simulink model "IRControlledSlidingDoor_Test"  (R2016a)
settings: Solver=ode3  SolverMode=SingleTasking  StartTime=0.0  StopTime=inf  FixedStep=0.1  RelTol=1e-3
libraries: arduinolib x7
settings Model: SimulationMode=external  ExtModeTrigDuration=2  Creator=Venkat  LastModifiedBy=venkatanchoori
settings DataIOCC: LimitDataPoints=on  SaveFormat=Array
settings OptimizationCC: ExpressionDepthLimit=2147483647  OptimizeModelRefInitCode=on  LifeSpan=1  MaxStackSize=64
settings DebuggingCC: UnderspecifiedInitializationDetection=Classic  MergeDetectMultiDrivingBlocksExec=none  StateNameClashWarn=warning
settings HardwareCC: ProdBitPerInt=16  ProdBitPerPointer=16  ProdLargestAtomicFloat=None  ProdWordSize=8  ProdHWDeviceType=Atmel->AVR
settings ModelReferenceCC: PropagateSignalLabelsOutOfModel=off
settings RTWCC: SystemTargetFile=ert.tlc  HardwareBoard=Arduino Mega 2560  TemplateMakefile=ert_default_tmf  GenerateReport=on  RTWVerbose=off  Toolchain=Arduino AVR v1.6.1  BuildConfiguration=Faster Runs  IncludeHyperlinkInReport=on  LaunchReport=on  GenerateTraceInfo=on  GenerateTraceReport=on  GenerateTraceReportSl=on  GenerateTraceReportSf=on  GenerateTraceReportEml=on
settings CodeAppCC: ForceParamTrailComments=on  IgnoreCustomStorageClasses=off  OperatorAnnotations=on  SimulinkDataObjDesc=on  SFDataObjDesc=on  MATLABFcnDesc=on  CustomSymbolStrType=$N$R$M  InsertBlockDesc=on  MATLABSourceComments=on  InternalIdentifier=Classic
settings ERTTargetCC: SupportContinuousTime=on  SupportVariableSizeSignals=on
settings ConfigComp: CovModelRefEnable=Off

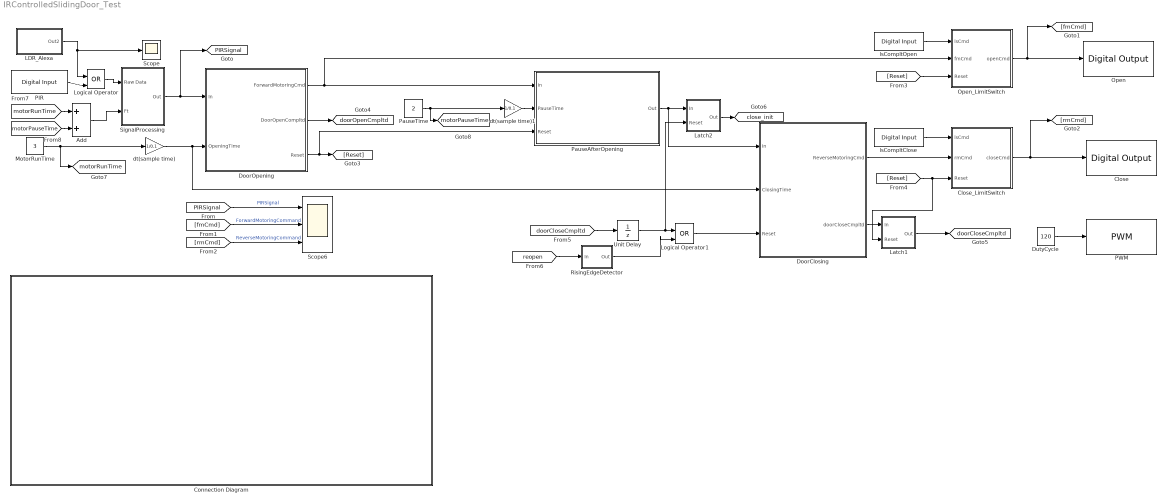
== system IRControlledSlidingDoor_Test ==
  Add : Sum
  Close : arduinolib/Digital Output  pinNumber=6  blockPlatform=arduino
  Close_LimitSwitch : Subsystem
  Connection Diagram : Subsystem  TreatAsAtomicUnit=on
      mask Display: image(imread('connectionDgm.png'));
  DoorClosing : Subsystem
      mask Display:
      | image(imread('GearReverse.JPG'));
      | port_label('input',1,'pauseCmpltd');
      | port_label('input',2,'ClosingTime');
      | port_label('input',3,'Reset');
      | % port_label('output',1,'fmCmd');
      | port_label('output',1,'rmCmd');
      | port_label('output',2,'doorCloseCmpltd');
  DoorOpening : Subsystem
      settings: RTWSystemCode=Nonreusable function  RTWFcnNameOpts=Use subsystem name  RTWFileNameOpts=Use subsystem name
      mask Display:
      | image(imread('GearForward.jpg'));
      | port_label('input',1,'PIRSignal');
      | port_label('input',2,'OpeningTime');
      | port_label('output',1,'fmCmd');
      | port_label('output',2,'DoorOpenCompltd');
      | port_label('output',3,'Reset');
  DutyCycle : Constant  Value=120
  LDR_Alexa : Subsystem
  Latch1 : Subsystem
  Latch2 : Subsystem
  Logical Operator : Logic  Operator=OR  IconShape=distinctive  AllPortsSameDT=off  OutDataTypeStr=boolean
  Logical Operator1 : Logic  Operator=OR  IconShape=distinctive  AllPortsSameDT=off  OutDataTypeStr=boolean
  MotorRunTime : Constant  Value=3
  Open : arduinolib/Digital Output  pinNumber=7  blockPlatform=arduino
  Open_LimitSwitch : Subsystem
  PIR : arduinolib/Digital Input  pinNumber=5  sampleTime=0.1  blockPlatform=arduino
  PWM : arduinolib/PWM  pinNumber=8  blockPlatform=arduino
  PauseAfterOpening : Subsystem
      mask Display:
      | image(imread('pause.JPG'));
      | port_label('input',1,'fmCmd');
      | port_label('input',2,'pauseTime');
      | port_label('input',3,'Reset');
      | % port_label('output',1,'fmCmd');
      | port_label('output',1,'PauseCmpltd');
  PauseTime : Constant  Value=2
  RisingEdgeDetector : Subsystem
  Scope : Scope
  Scope6 : Scope  NumInputPorts=3
  SignalProcessing : Subsystem
  Unit Delay : UnitDelay  SampleTime=-1
  dt(sample time) : Gain  Gain=1/0.1
  dt(sample time)1 : Gain  Gain=1/0.1
  lsCompltClose : arduinolib/Digital Input  pinNumber=3  sampleTime=0.1  blockPlatform=arduino
  lsCompltOpen : arduinolib/Digital Input  pinNumber=2  sampleTime=0.1  blockPlatform=arduino
  tag scope: PIRSignal=global, close_init=global, doorCloseCmpltd=global, doorOpenCmpltd=global, motorPauseTime=global, motorRunTime=global
  wires:
  PauseTime/1 -> [motorPauseTime], dt(sample time)1/1
  SignalProcessing/1(Out) -> [PIRSignal], DoorOpening/1(In)
  DoorOpening/3(Reset) -> PauseAfterOpening/3(Reset), [Reset]
  PauseAfterOpening/1(Out) -> DoorClosing/1(In), Latch2/1(In)
  DoorClosing/1(ReverseMotoringCmd) -> Close_LimitSwitch/2(rmCmd)
  [PIRSignal] -> Scope6/1  "PIRSignal"
  [fmCmd] -> Scope6/2  "ForwardMotoringCommand"
  [rmCmd] -> Scope6/3  "ReverseMotoringCommand"
  DoorOpening/1(ForwardMotoringCmd) -> Open_LimitSwitch/2(fmCmd), PauseAfterOpening/1(In)
  Close_LimitSwitch/1(closeCmd) -> Close/1, [rmCmd]
  lsCompltOpen/1 -> Open_LimitSwitch/1(lsCmd)
  Open_LimitSwitch/1(openCmd) -> Open/1, [fmCmd]
  [Reset] -> Open_LimitSwitch/3(Reset)
  lsCompltClose/1 -> Close_LimitSwitch/1(lsCmd)
  DoorOpening/2(DoorOpenCompltd) -> [doorOpenCmpltd]
  dt(sample time)/1 -> DoorClosing/2(ClosingTime), DoorOpening/2(OpeningTime)
  dt(sample time)1/1 -> PauseAfterOpening/2(PauseTime)
  [doorCloseCmpltd] -> Unit Delay/1
  Latch2/1(Out) -> [close_init]
  Unit Delay/1 -> Logical Operator1/1, Latch2/2(Reset)
  Latch1/1(Out) -> [doorCloseCmpltd]
  DoorClosing/2(doorCloseCmpltd) -> Latch1/1(In)
  [Reset] -> Latch1/2(Reset), Close_LimitSwitch/3(Reset)
  [reopen] -> RisingEdgeDetector/1(In)
  Logical Operator1/1 -> DoorClosing/3(Reset)
  RisingEdgeDetector/1(Out) -> Logical Operator1/2
  MotorRunTime/1 -> [motorRunTime], dt(sample time)/1
  [motorRunTime] -> Add/1
  [motorPauseTime] -> Add/2
  Add/1 -> SignalProcessing/2(Ft)
  DutyCycle/1 -> PWM/1
  PIR/1 -> Logical Operator/2
  Logical Operator/1 -> SignalProcessing/1(Raw Data)
  LDR_Alexa/1(Out2) -> Scope/1, Logical Operator/1

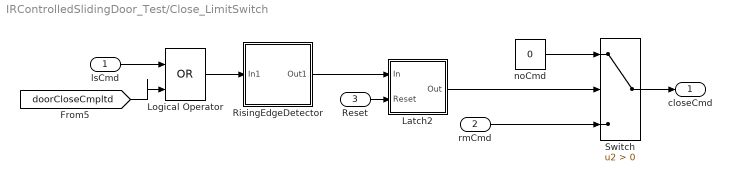
== system IRControlledSlidingDoor_Test/Close_LimitSwitch ==
  lsCmd : Inport
  rmCmd : Inport  Port=2
  Reset : Inport  Port=3
  Latch2 : Subsystem
  Logical Operator : Logic  Operator=OR  IconShape=distinctive  AllPortsSameDT=off  OutDataTypeStr=boolean
  RisingEdgeDetector : Subsystem
  Switch : Switch  Criteria=u2 > Threshold
  noCmd : Constant  Value=0
  closeCmd : Outport
  wires:
  noCmd/1 -> Switch/1
  Latch2/1(Out) -> Switch/2
  Switch/1 -> closeCmd/1
  RisingEdgeDetector/1(Out1) -> Latch2/1(In)
  Reset/1 -> Latch2/2(Reset)
  rmCmd/1 -> Switch/3
  lsCmd/1 -> Logical Operator/1
  Logical Operator/1 -> RisingEdgeDetector/1(In1)
  [doorCloseCmpltd] -> Logical Operator/2

== system IRControlledSlidingDoor_Test/Connection Diagram ==

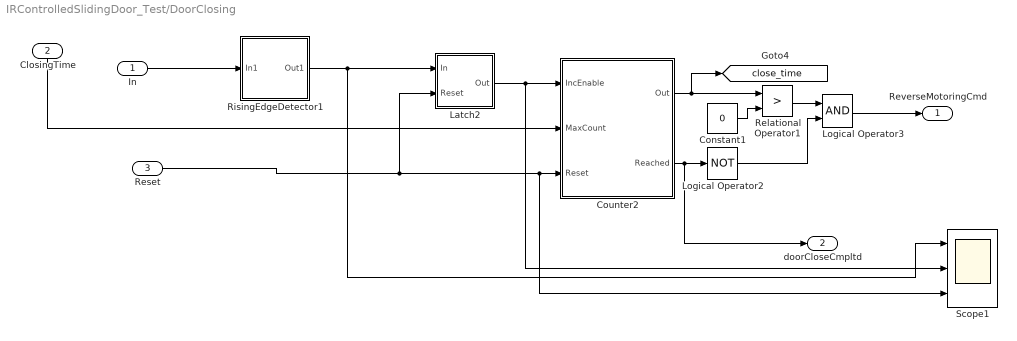
== system IRControlledSlidingDoor_Test/DoorClosing ==
  In : Inport
  ClosingTime : Inport  Port=2
  Reset : Inport  Port=3
  Constant1 : Constant  Value=0
  Counter2 : Subsystem
  Latch2 : Subsystem
  Logical Operator2 : Logic  Operator=NOT  AllPortsSameDT=off  OutDataTypeStr=boolean
  Logical Operator3 : Logic  AllPortsSameDT=off  OutDataTypeStr=boolean
  Relational Operator1 : RelationalOperator  Operator=>  OutDataTypeStr=boolean
  RisingEdgeDetector1 : Subsystem
  Scope1 : Scope  NumInputPorts=3
  ReverseMotoringCmd : Outport
  doorCloseCmpltd : Outport  Port=2
  tag scope: close_time=global
  wires:
  ClosingTime/1 -> Counter2/2(MaxCount)
  Logical Operator3/1 -> ReverseMotoringCmd/1
  Reset/1 -> Latch2/2(Reset), Scope1/3, Counter2/3(Reset)
  In/1 -> RisingEdgeDetector1/1(In1)
  Constant1/1 -> Relational Operator1/2
  Logical Operator2/1 -> Logical Operator3/2
  Latch2/1(Out) -> Scope1/2, Counter2/1(IncEnable)
  Counter2/1(Out) -> [close_time], Relational Operator1/1
  Relational Operator1/1 -> Logical Operator3/1
  Counter2/2(Reached) -> doorCloseCmpltd/1, Logical Operator2/1
  RisingEdgeDetector1/1(Out1) -> Scope1/1, Latch2/1(In)

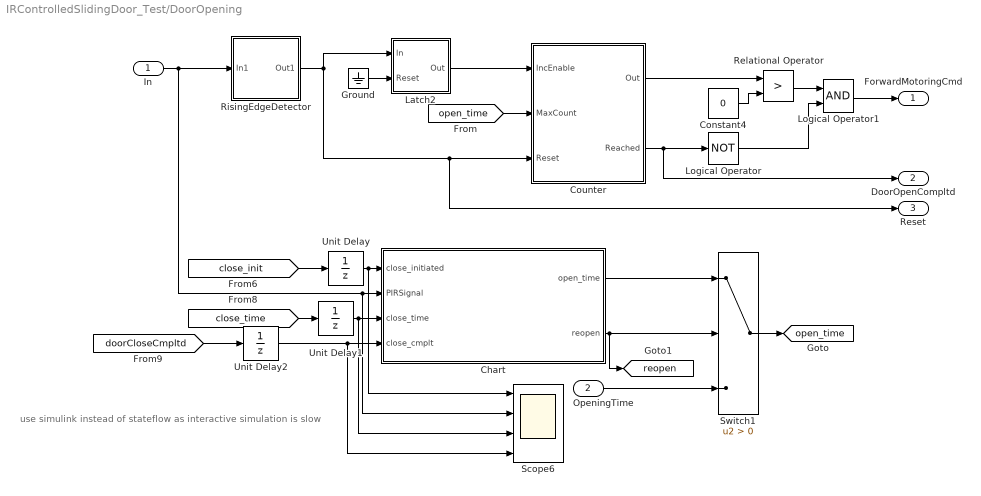
== system IRControlledSlidingDoor_Test/DoorOpening ==
  note: use simulink instead of stateflow as interactive simulation is slow
  In : Inport
  OpeningTime : Inport  Port=2
  Chart : Stateflow chart  TreatAsAtomicUnit=on
  Constant4 : Constant  Value=0
  Counter : Subsystem
  Ground : Ground
  Latch2 : Subsystem
  Logical Operator : Logic  Operator=NOT  AllPortsSameDT=off  OutDataTypeStr=boolean
  Logical Operator1 : Logic  AllPortsSameDT=off  OutDataTypeStr=boolean
  Relational Operator : RelationalOperator  Operator=>  OutDataTypeStr=boolean
  RisingEdgeDetector : Subsystem
  Scope6 : Scope  NumInputPorts=4
  Switch1 : Switch  Criteria=u2 > Threshold
  Unit Delay : UnitDelay  SampleTime=-1
  Unit Delay1 : UnitDelay  SampleTime=-1
  Unit Delay2 : UnitDelay  SampleTime=-1
  ForwardMotoringCmd : Outport
  DoorOpenCompltd : Outport  Port=2
  Reset : Outport  Port=3
  tag scope: open_time=global, reopen=global
  wires:
  Ground/1 -> Latch2/2(Reset)
  Logical Operator1/1 -> ForwardMotoringCmd/1
  RisingEdgeDetector/1(Out1) -> Counter/3(Reset), Reset/1, Latch2/1(In)
  Constant4/1 -> Relational Operator/2
  Latch2/1(Out) -> Counter/1(IncEnable)
  Logical Operator/1 -> Logical Operator1/2
  Counter/2(Reached) -> DoorOpenCompltd/1, Logical Operator/1
  Relational Operator/1 -> Logical Operator1/1
  Counter/1(Out) -> Relational Operator/1
  [close_init] -> Unit Delay/1
  [close_time] -> Unit Delay1/1
  [doorCloseCmpltd] -> Unit Delay2/1
  OpeningTime/1 -> Switch1/3
  Chart/2(reopen) -> Switch1/2, [reopen]
  Chart/1(open_time) -> Switch1/1
  Switch1/1 -> [open_time]
  [open_time] -> Counter/2(MaxCount)
  Unit Delay1/1 -> Scope6/3, Chart/3(close_time)
  Unit Delay2/1 -> Scope6/4, Chart/4(close_cmplt)
  Unit Delay/1 -> Scope6/1, Chart/1(close_initiated)
  In/1 -> Scope6/2, Chart/2(PIRSignal), RisingEdgeDetector/1(In1)

== system IRControlledSlidingDoor_Test/LDR_Alexa ==
  Analog Input : arduinolib/Analog Input  pinNumber=0  sampleTime=1  blockPlatform=arduino
  Constant : Constant  Value=100
  Relational Operator : RelationalOperator  OutDataTypeStr=boolean
  Scope : Scope  NumInputPorts=2
  Out2 : Outport
  wires:
  Analog Input/1 -> Scope/1, Relational Operator/1
  Relational Operator/1 -> Scope/2, Out2/1
  Constant/1 -> Relational Operator/2

== system IRControlledSlidingDoor_Test/Latch1 ==
  In : Inport
  Reset : Inport  Port=2
  Constant1 : Constant  Value=0  OutDataTypeStr=boolean
  Switch1 : Switch  Criteria=u2 > Threshold
  Switch2 : Switch  Criteria=u2 > Threshold
  Unit Delay2 : UnitDelay  SampleTime=-1
  Out : Outport
  wires:
  Unit Delay2/1 -> Switch2/3
  Switch2/1 -> Switch1/3
  In/1 -> Switch2/1, Switch2/2
  Switch1/1 -> Unit Delay2/1, Out/1
  Constant1/1 -> Switch1/1
  Reset/1 -> Switch1/2

== system IRControlledSlidingDoor_Test/Latch2 ==
  In : Inport
  Reset : Inport  Port=2
  Constant1 : Constant  Value=0  OutDataTypeStr=boolean
  Switch1 : Switch  Criteria=u2 > Threshold
  Switch2 : Switch  Criteria=u2 > Threshold
  Unit Delay2 : UnitDelay  SampleTime=-1
  Out : Outport
  wires:
  Unit Delay2/1 -> Switch2/3
  Switch2/1 -> Switch1/3
  In/1 -> Switch2/1, Switch2/2
  Switch1/1 -> Unit Delay2/1, Out/1
  Constant1/1 -> Switch1/1
  Reset/1 -> Switch1/2

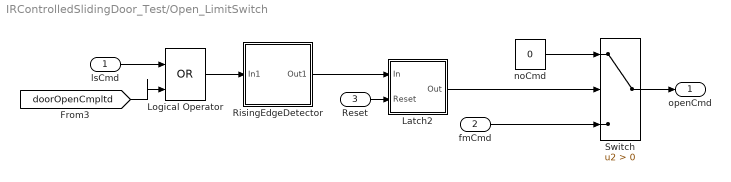
== system IRControlledSlidingDoor_Test/Open_LimitSwitch ==
  lsCmd : Inport
  fmCmd : Inport  Port=2
  Reset : Inport  Port=3
  Latch2 : Subsystem
  Logical Operator : Logic  Operator=OR  IconShape=distinctive  AllPortsSameDT=off  OutDataTypeStr=boolean
  RisingEdgeDetector : Subsystem
  Switch : Switch  Criteria=u2 > Threshold
  noCmd : Constant  Value=0
  openCmd : Outport
  wires:
  noCmd/1 -> Switch/1
  Latch2/1(Out) -> Switch/2
  Switch/1 -> openCmd/1
  RisingEdgeDetector/1(Out1) -> Latch2/1(In)
  Reset/1 -> Latch2/2(Reset)
  fmCmd/1 -> Switch/3
  lsCmd/1 -> Logical Operator/1
  Logical Operator/1 -> RisingEdgeDetector/1(In1)
  [doorOpenCmpltd] -> Logical Operator/2

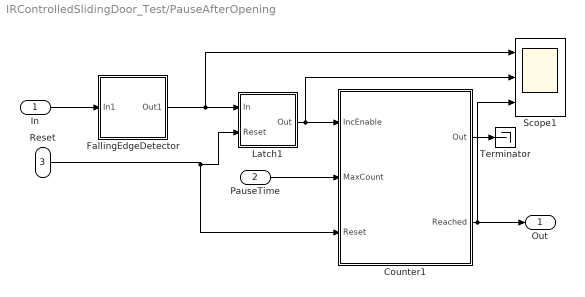
== system IRControlledSlidingDoor_Test/PauseAfterOpening ==
  In : Inport
  PauseTime : Inport  Port=2
  Reset : Inport  Port=3
  Counter1 : Subsystem
  FallingEdgeDetector : Subsystem
  Latch1 : Subsystem
  Scope1 : Scope  NumInputPorts=3
  Terminator : Terminator
  Out : Outport
  wires:
  Reset/1 -> Counter1/3(Reset), Latch1/2(Reset)
  FallingEdgeDetector/1(Out1) -> Scope1/1, Latch1/1(In)
  Latch1/1(Out) -> Scope1/2, Counter1/1(IncEnable)
  PauseTime/1 -> Counter1/2(MaxCount)
  Counter1/2(Reached) -> Out/1, Scope1/3
  In/1 -> FallingEdgeDetector/1(In1)
  Counter1/1(Out) -> Terminator/1

== system IRControlledSlidingDoor_Test/RisingEdgeDetector ==
  In : Inport
  Logical Operator1 : Logic  Operator=NOT  AllPortsSameDT=off  OutDataTypeStr=boolean
  Logical Operator4 : Logic  AllPortsSameDT=off  OutDataTypeStr=boolean
  Unit Delay : UnitDelay  SampleTime=-1
  Out : Outport
  wires:
  Unit Delay/1 -> Logical Operator1/1
  Logical Operator4/1 -> Out/1
  In/1 -> Logical Operator4/1, Unit Delay/1
  Logical Operator1/1 -> Logical Operator4/2

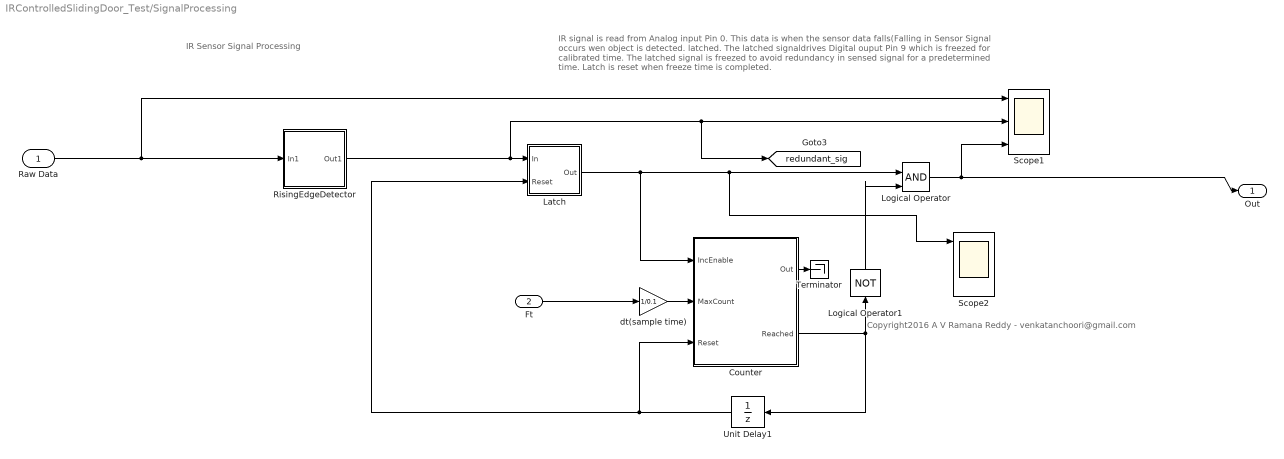
== system IRControlledSlidingDoor_Test/SignalProcessing ==
  note: IR signal is read from Analog input Pin 0. This data is when the sensor data falls(Falling in Sensor Signal
      |  occurs wen object is detected. latched. The latched signaldrives Digital ouput Pin 9 which is freezed for
      | calibrated time. The latched signal is freezed to avoid redundancy in sensed signal for a predetermined time.
      | Latch is reset when freeze time is completed.
  note: Copyright2016 A V Ramana Reddy - venkatanchoori@gmail.com
  note: IR Sensor Signal Processing
  Raw Data : Inport
  Ft : Inport  Port=2
  Counter : Subsystem
  Latch : Subsystem
  Logical Operator : Logic  IconShape=distinctive  AllPortsSameDT=off  OutDataTypeStr=boolean
  Logical Operator1 : Logic  Operator=NOT  IconShape=distinctive  AllPortsSameDT=off  OutDataTypeStr=boolean
  RisingEdgeDetector : Subsystem
  Scope1 : Scope  NumInputPorts=3
  Scope2 : Scope  NumInputPorts=3
  Terminator : Terminator
  Unit Delay1 : UnitDelay  SampleTime=-1
  dt(sample time) : Gain  Gain=1/0.1
  Out : Outport
  tag scope: redundant_sig=global
  wires:
  RisingEdgeDetector/1(Out1) -> Latch/1(In), [redundant_sig], Scope1/2
  Latch/1(Out) -> Counter/1(IncEnable), Scope2/1, Logical Operator/1
  Ft/1 -> dt(sample time)/1
  Counter/2(Reached) -> Unit Delay1/1, Logical Operator1/1
  Counter/1(Out) -> Terminator/1
  Unit Delay1/1 -> Counter/3(Reset), Latch/2(Reset)
  Logical Operator/1 -> Out/1, Scope1/3
  Logical Operator1/1 -> Logical Operator/2
  dt(sample time)/1 -> Counter/2(MaxCount)
  Raw Data/1 -> Scope1/1, RisingEdgeDetector/1(In1)

== system IRControlledSlidingDoor_Test/Close_LimitSwitch/Latch2 ==
  In : Inport
  Reset : Inport  Port=2
  Constant1 : Constant  Value=0  OutDataTypeStr=boolean
  Switch1 : Switch  Criteria=u2 > Threshold
  Switch2 : Switch  Criteria=u2 > Threshold
  Unit Delay2 : UnitDelay  SampleTime=-1
  Out : Outport
  wires:
  Unit Delay2/1 -> Switch2/3
  Switch2/1 -> Switch1/3
  In/1 -> Switch2/1, Switch2/2
  Switch1/1 -> Unit Delay2/1, Out/1
  Constant1/1 -> Switch1/1
  Reset/1 -> Switch1/2

== system IRControlledSlidingDoor_Test/Close_LimitSwitch/RisingEdgeDetector ==
  In1 : Inport
  Logical Operator1 : Logic  Operator=NOT  AllPortsSameDT=off  OutDataTypeStr=boolean
  Logical Operator4 : Logic  AllPortsSameDT=off  OutDataTypeStr=boolean
  Unit Delay : UnitDelay  SampleTime=-1
  Out1 : Outport
  wires:
  Unit Delay/1 -> Logical Operator1/1
  Logical Operator4/1 -> Out1/1
  In1/1 -> Logical Operator4/1, Unit Delay/1
  Logical Operator1/1 -> Logical Operator4/2

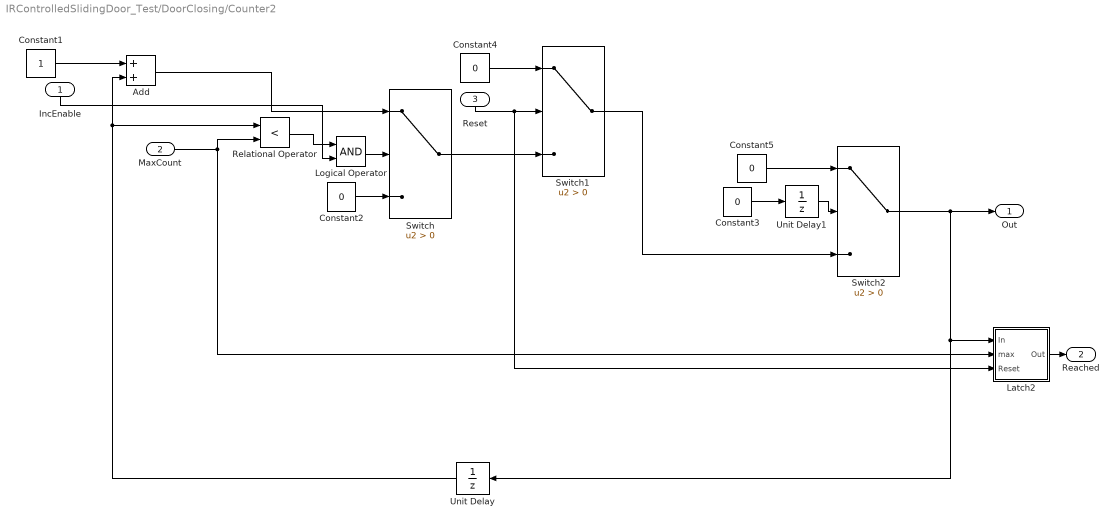
== system IRControlledSlidingDoor_Test/DoorClosing/Counter2 ==
  IncEnable : Inport
  MaxCount : Inport  Port=2
  Reset : Inport  Port=3
  Add : Sum
  Constant1 : Constant
  Constant{2..5} (4 alike) : Constant  Value=0
  Latch2 : Subsystem
  Logical Operator : Logic  AllPortsSameDT=off  OutDataTypeStr=boolean
  Relational Operator : RelationalOperator  Operator=<  OutDataTypeStr=boolean
  Switch : Switch  Criteria=u2 > Threshold
  Switch1 : Switch  Criteria=u2 > Threshold
  Switch2 : Switch  Criteria=u2 > Threshold
  Unit Delay : UnitDelay  SampleTime=-1
  Unit Delay1 : UnitDelay  InitialCondition=1  SampleTime=-1
  Out : Outport
  Reached : Outport  Port=2
  wires:
  Logical Operator/1 -> Switch/2
  Relational Operator/1 -> Logical Operator/1
  Add/1 -> Switch/1
  Constant1/1 -> Add/1
  Constant2/1 -> Switch/3
  Unit Delay/1 -> Relational Operator/1, Add/2
  Switch/1 -> Switch1/3
  Reset/1 -> Latch2/3(Reset), Switch1/2
  Latch2/1(Out) -> Reached/1
  Constant3/1 -> Unit Delay1/1
  Constant4/1 -> Switch1/1
  Unit Delay1/1 -> Switch2/2
  Constant5/1 -> Switch2/1
  Switch1/1 -> Switch2/3
  Switch2/1 -> Latch2/1(In), Unit Delay/1, Out/1
  IncEnable/1 -> Logical Operator/2
  MaxCount/1 -> Relational Operator/2, Latch2/2(max)

== system IRControlledSlidingDoor_Test/DoorClosing/Latch2 ==
  In : Inport
  Reset : Inport  Port=2
  Constant1 : Constant  Value=0  OutDataTypeStr=boolean
  Switch1 : Switch  Criteria=u2 > Threshold
  Switch2 : Switch  Criteria=u2 > Threshold
  Unit Delay2 : UnitDelay  SampleTime=-1
  Out : Outport
  wires:
  Unit Delay2/1 -> Switch2/3
  Switch2/1 -> Switch1/3
  In/1 -> Switch2/1, Switch2/2
  Switch1/1 -> Unit Delay2/1, Out/1
  Constant1/1 -> Switch1/1
  Reset/1 -> Switch1/2

== system IRControlledSlidingDoor_Test/DoorClosing/RisingEdgeDetector1 ==
  In1 : Inport
  Logical Operator1 : Logic  Operator=NOT  AllPortsSameDT=off  OutDataTypeStr=boolean
  Logical Operator4 : Logic  AllPortsSameDT=off  OutDataTypeStr=boolean
  Unit Delay : UnitDelay  SampleTime=-1
  Out1 : Outport
  wires:
  Unit Delay/1 -> Logical Operator1/1
  Logical Operator4/1 -> Out1/1
  In1/1 -> Logical Operator4/1, Unit Delay/1
  Logical Operator1/1 -> Logical Operator4/2

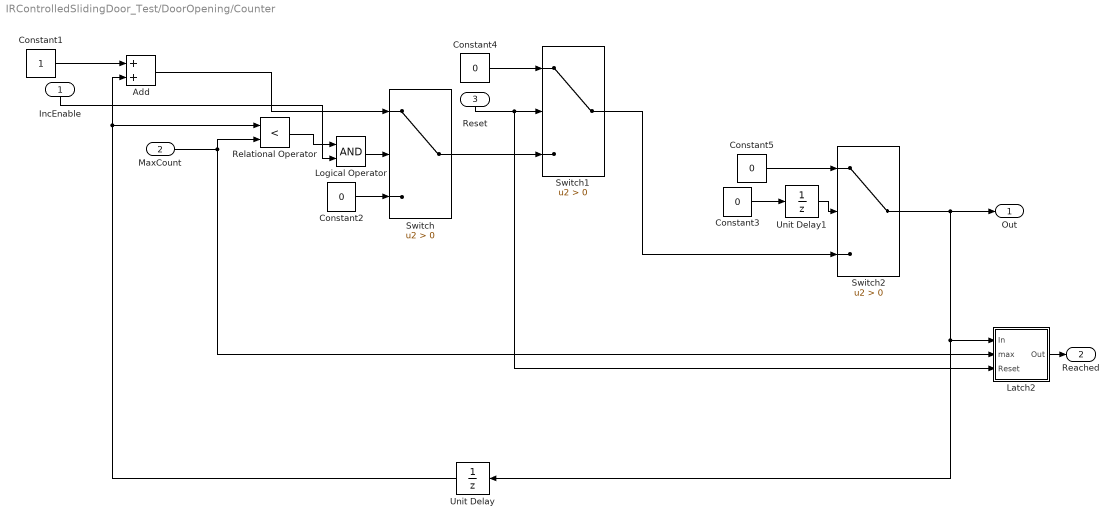
== system IRControlledSlidingDoor_Test/DoorOpening/Counter ==
  IncEnable : Inport
  MaxCount : Inport  Port=2
  Reset : Inport  Port=3
  Add : Sum
  Constant1 : Constant
  Constant{2..5} (4 alike) : Constant  Value=0
  Latch2 : Subsystem
  Logical Operator : Logic  AllPortsSameDT=off  OutDataTypeStr=boolean
  Relational Operator : RelationalOperator  Operator=<  OutDataTypeStr=boolean
  Switch : Switch  Criteria=u2 > Threshold
  Switch1 : Switch  Criteria=u2 > Threshold
  Switch2 : Switch  Criteria=u2 > Threshold
  Unit Delay : UnitDelay  SampleTime=-1
  Unit Delay1 : UnitDelay  InitialCondition=1  SampleTime=-1
  Out : Outport
  Reached : Outport  Port=2
  wires:
  Logical Operator/1 -> Switch/2
  Relational Operator/1 -> Logical Operator/1
  Add/1 -> Switch/1
  Constant1/1 -> Add/1
  Constant2/1 -> Switch/3
  Unit Delay/1 -> Relational Operator/1, Add/2
  Switch/1 -> Switch1/3
  Reset/1 -> Latch2/3(Reset), Switch1/2
  Latch2/1(Out) -> Reached/1
  Constant3/1 -> Unit Delay1/1
  Constant4/1 -> Switch1/1
  Unit Delay1/1 -> Switch2/2
  Constant5/1 -> Switch2/1
  Switch1/1 -> Switch2/3
  Switch2/1 -> Latch2/1(In), Unit Delay/1, Out/1
  IncEnable/1 -> Logical Operator/2
  MaxCount/1 -> Relational Operator/2, Latch2/2(max)

== system IRControlledSlidingDoor_Test/DoorOpening/Latch2 ==
  In : Inport
  Reset : Inport  Port=2
  Constant1 : Constant  Value=0  OutDataTypeStr=boolean
  Switch1 : Switch  Criteria=u2 > Threshold
  Switch2 : Switch  Criteria=u2 > Threshold
  Unit Delay2 : UnitDelay  SampleTime=-1
  Out : Outport
  wires:
  Unit Delay2/1 -> Switch2/3
  Switch2/1 -> Switch1/3
  In/1 -> Switch2/1, Switch2/2
  Switch1/1 -> Unit Delay2/1, Out/1
  Constant1/1 -> Switch1/1
  Reset/1 -> Switch1/2

== system IRControlledSlidingDoor_Test/DoorOpening/RisingEdgeDetector ==
  In1 : Inport
  Logical Operator1 : Logic  Operator=NOT  AllPortsSameDT=off  OutDataTypeStr=boolean
  Logical Operator4 : Logic  AllPortsSameDT=off  OutDataTypeStr=boolean
  Unit Delay : UnitDelay  SampleTime=-1
  Out1 : Outport
  wires:
  Unit Delay/1 -> Logical Operator1/1
  Logical Operator4/1 -> Out1/1
  In1/1 -> Logical Operator4/1, Unit Delay/1
  Logical Operator1/1 -> Logical Operator4/2

== system IRControlledSlidingDoor_Test/Open_LimitSwitch/Latch2 ==
  In : Inport
  Reset : Inport  Port=2
  Constant1 : Constant  Value=0  OutDataTypeStr=boolean
  Switch1 : Switch  Criteria=u2 > Threshold
  Switch2 : Switch  Criteria=u2 > Threshold
  Unit Delay2 : UnitDelay  SampleTime=-1
  Out : Outport
  wires:
  Unit Delay2/1 -> Switch2/3
  Switch2/1 -> Switch1/3
  In/1 -> Switch2/1, Switch2/2
  Switch1/1 -> Unit Delay2/1, Out/1
  Constant1/1 -> Switch1/1
  Reset/1 -> Switch1/2

== system IRControlledSlidingDoor_Test/Open_LimitSwitch/RisingEdgeDetector ==
  In1 : Inport
  Logical Operator1 : Logic  Operator=NOT  AllPortsSameDT=off  OutDataTypeStr=boolean
  Logical Operator4 : Logic  AllPortsSameDT=off  OutDataTypeStr=boolean
  Unit Delay : UnitDelay  SampleTime=-1
  Out1 : Outport
  wires:
  Unit Delay/1 -> Logical Operator1/1
  Logical Operator4/1 -> Out1/1
  In1/1 -> Logical Operator4/1, Unit Delay/1
  Logical Operator1/1 -> Logical Operator4/2

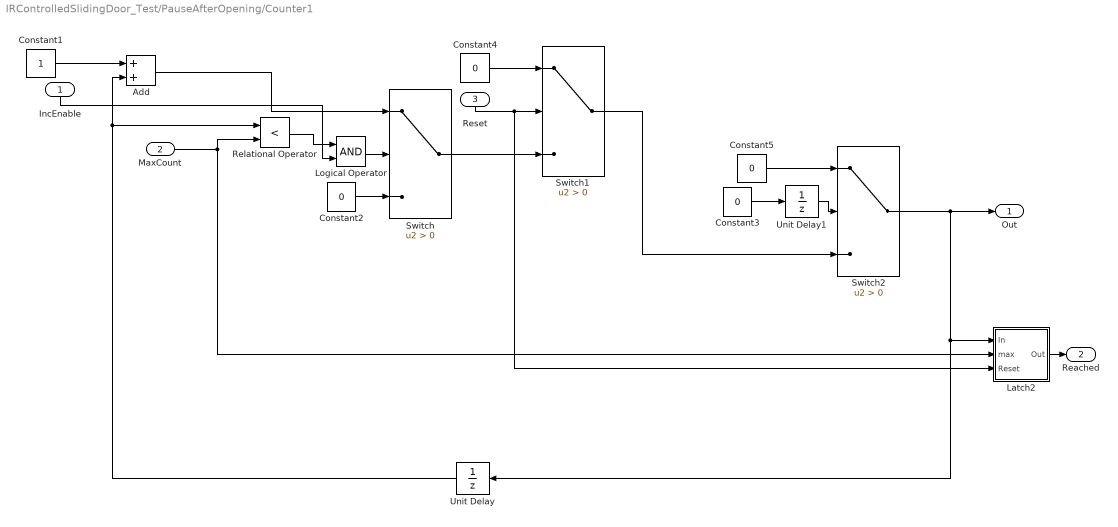
== system IRControlledSlidingDoor_Test/PauseAfterOpening/Counter1 ==
  IncEnable : Inport
  MaxCount : Inport  Port=2
  Reset : Inport  Port=3
  Add : Sum
  Constant1 : Constant
  Constant{2..5} (4 alike) : Constant  Value=0
  Latch2 : Subsystem
  Logical Operator : Logic  AllPortsSameDT=off  OutDataTypeStr=boolean
  Relational Operator : RelationalOperator  Operator=<  OutDataTypeStr=boolean
  Switch : Switch  Criteria=u2 > Threshold
  Switch1 : Switch  Criteria=u2 > Threshold
  Switch2 : Switch  Criteria=u2 > Threshold
  Unit Delay : UnitDelay  SampleTime=-1
  Unit Delay1 : UnitDelay  InitialCondition=1  SampleTime=-1
  Out : Outport
  Reached : Outport  Port=2
  wires:
  Logical Operator/1 -> Switch/2
  Relational Operator/1 -> Logical Operator/1
  Add/1 -> Switch/1
  Constant1/1 -> Add/1
  Constant2/1 -> Switch/3
  Unit Delay/1 -> Relational Operator/1, Add/2
  Switch/1 -> Switch1/3
  Reset/1 -> Latch2/3(Reset), Switch1/2
  Latch2/1(Out) -> Reached/1
  Constant3/1 -> Unit Delay1/1
  Constant4/1 -> Switch1/1
  Unit Delay1/1 -> Switch2/2
  Constant5/1 -> Switch2/1
  Switch1/1 -> Switch2/3
  Switch2/1 -> Latch2/1(In), Unit Delay/1, Out/1
  IncEnable/1 -> Logical Operator/2
  MaxCount/1 -> Relational Operator/2, Latch2/2(max)

== system IRControlledSlidingDoor_Test/PauseAfterOpening/FallingEdgeDetector ==
  In1 : Inport
  Logical Operator4 : Logic  AllPortsSameDT=off  OutDataTypeStr=boolean
  Logical Operator7 : Logic  Operator=NOT  AllPortsSameDT=off  OutDataTypeStr=boolean
  Unit Delay : UnitDelay  SampleTime=-1
  Out1 : Outport
  wires:
  In1/1 -> Unit Delay/1, Logical Operator7/1
  Unit Delay/1 -> Logical Operator4/2
  Logical Operator4/1 -> Out1/1
  Logical Operator7/1 -> Logical Operator4/1

== system IRControlledSlidingDoor_Test/PauseAfterOpening/Latch1 ==
  In : Inport
  Reset : Inport  Port=2
  Constant1 : Constant  Value=0  OutDataTypeStr=boolean
  Switch1 : Switch  Criteria=u2 > Threshold
  Switch2 : Switch  Criteria=u2 > Threshold
  Unit Delay2 : UnitDelay  SampleTime=-1
  Out : Outport
  wires:
  Unit Delay2/1 -> Switch2/3
  Switch2/1 -> Switch1/3
  In/1 -> Switch2/1, Switch2/2
  Switch1/1 -> Unit Delay2/1, Out/1
  Constant1/1 -> Switch1/1
  Reset/1 -> Switch1/2

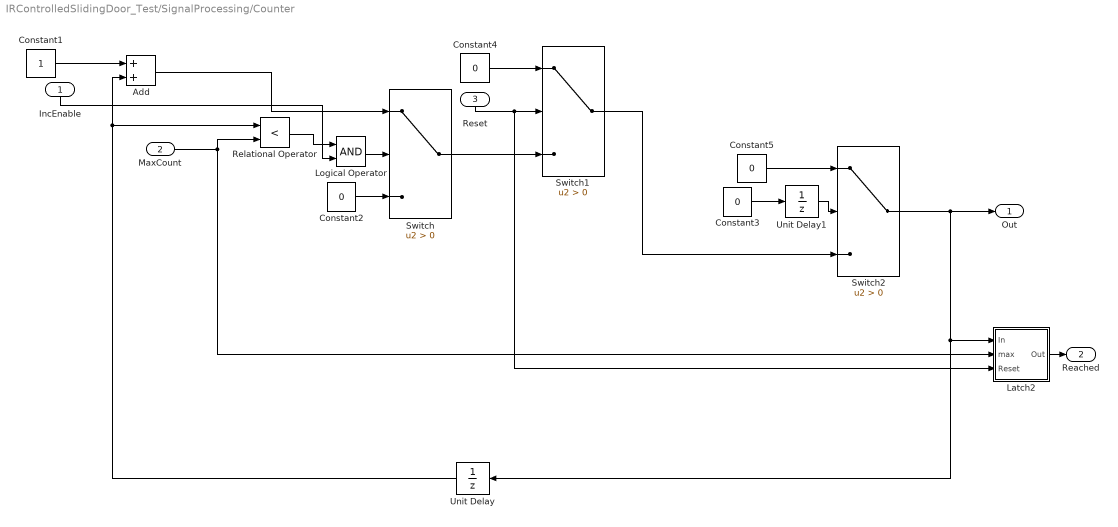
== system IRControlledSlidingDoor_Test/SignalProcessing/Counter ==
  IncEnable : Inport
  MaxCount : Inport  Port=2
  Reset : Inport  Port=3
  Add : Sum
  Constant1 : Constant
  Constant{2..5} (4 alike) : Constant  Value=0
  Latch2 : Subsystem
  Logical Operator : Logic  AllPortsSameDT=off  OutDataTypeStr=boolean
  Relational Operator : RelationalOperator  Operator=<  OutDataTypeStr=boolean
  Switch : Switch  Criteria=u2 > Threshold
  Switch1 : Switch  Criteria=u2 > Threshold
  Switch2 : Switch  Criteria=u2 > Threshold
  Unit Delay : UnitDelay  SampleTime=-1
  Unit Delay1 : UnitDelay  InitialCondition=1  SampleTime=-1
  Out : Outport
  Reached : Outport  Port=2
  wires:
  Logical Operator/1 -> Switch/2
  Relational Operator/1 -> Logical Operator/1
  Add/1 -> Switch/1
  Constant1/1 -> Add/1
  Constant2/1 -> Switch/3
  Unit Delay/1 -> Relational Operator/1, Add/2
  Switch/1 -> Switch1/3
  Reset/1 -> Latch2/3(Reset), Switch1/2
  Latch2/1(Out) -> Reached/1
  Constant3/1 -> Unit Delay1/1
  Constant4/1 -> Switch1/1
  Unit Delay1/1 -> Switch2/2
  Constant5/1 -> Switch2/1
  Switch1/1 -> Switch2/3
  Switch2/1 -> Latch2/1(In), Unit Delay/1, Out/1
  IncEnable/1 -> Logical Operator/2
  MaxCount/1 -> Relational Operator/2, Latch2/2(max)

== system IRControlledSlidingDoor_Test/SignalProcessing/Latch ==
  In : Inport
  Reset : Inport  Port=2
  Constant1 : Constant  Value=0  OutDataTypeStr=boolean
  Switch1 : Switch  Criteria=u2 > Threshold
  Switch2 : Switch  Criteria=u2 > Threshold
  Unit Delay2 : UnitDelay  SampleTime=-1
  Out : Outport
  wires:
  Unit Delay2/1 -> Switch2/3
  Switch2/1 -> Switch1/3
  In/1 -> Switch2/1, Switch2/2
  Switch1/1 -> Unit Delay2/1, Out/1
  Constant1/1 -> Switch1/1
  Reset/1 -> Switch1/2

== system IRControlledSlidingDoor_Test/SignalProcessing/RisingEdgeDetector ==
  In1 : Inport
  Logical Operator1 : Logic  Operator=NOT  AllPortsSameDT=off  OutDataTypeStr=boolean
  Logical Operator4 : Logic  AllPortsSameDT=off  OutDataTypeStr=boolean
  Unit Delay : UnitDelay  SampleTime=-1
  Out1 : Outport
  wires:
  Unit Delay/1 -> Logical Operator1/1
  Logical Operator4/1 -> Out1/1
  In1/1 -> Logical Operator4/1, Unit Delay/1
  Logical Operator1/1 -> Logical Operator4/2

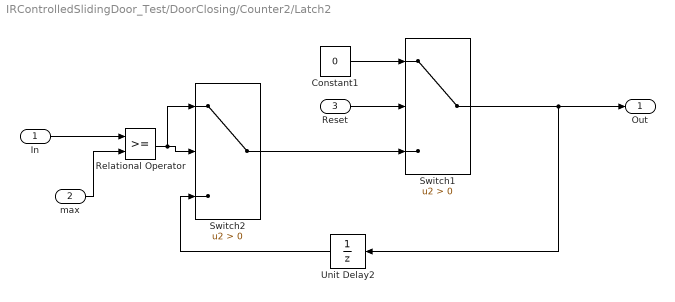
== system IRControlledSlidingDoor_Test/DoorClosing/Counter2/Latch2 ==
  In : Inport
  max : Inport  Port=2
  Reset : Inport  Port=3
  Constant1 : Constant  Value=0  OutDataTypeStr=boolean
  Relational Operator : RelationalOperator  OutDataTypeStr=boolean
  Switch1 : Switch  Criteria=u2 > Threshold
  Switch2 : Switch  Criteria=u2 > Threshold
  Unit Delay2 : UnitDelay  SampleTime=-1
  Out : Outport
  wires:
  Unit Delay2/1 -> Switch2/3
  Switch2/1 -> Switch1/3
  Switch1/1 -> Unit Delay2/1, Out/1
  Constant1/1 -> Switch1/1
  Reset/1 -> Switch1/2
  In/1 -> Relational Operator/1
  Relational Operator/1 -> Switch2/1, Switch2/2
  max/1 -> Relational Operator/2

== system IRControlledSlidingDoor_Test/DoorOpening/Counter/Latch2 ==
  In : Inport
  max : Inport  Port=2
  Reset : Inport  Port=3
  Constant1 : Constant  Value=0  OutDataTypeStr=boolean
  Relational Operator : RelationalOperator  OutDataTypeStr=boolean
  Switch1 : Switch  Criteria=u2 > Threshold
  Switch2 : Switch  Criteria=u2 > Threshold
  Unit Delay2 : UnitDelay  SampleTime=-1
  Out : Outport
  wires:
  Unit Delay2/1 -> Switch2/3
  Switch2/1 -> Switch1/3
  Switch1/1 -> Unit Delay2/1, Out/1
  Constant1/1 -> Switch1/1
  Reset/1 -> Switch1/2
  In/1 -> Relational Operator/1
  Relational Operator/1 -> Switch2/1, Switch2/2
  max/1 -> Relational Operator/2

== system IRControlledSlidingDoor_Test/PauseAfterOpening/Counter1/Latch2 ==
  In : Inport
  max : Inport  Port=2
  Reset : Inport  Port=3
  Constant1 : Constant  Value=0  OutDataTypeStr=boolean
  Relational Operator : RelationalOperator  OutDataTypeStr=boolean
  Switch1 : Switch  Criteria=u2 > Threshold
  Switch2 : Switch  Criteria=u2 > Threshold
  Unit Delay2 : UnitDelay  SampleTime=-1
  Out : Outport
  wires:
  Unit Delay2/1 -> Switch2/3
  Switch2/1 -> Switch1/3
  Switch1/1 -> Unit Delay2/1, Out/1
  Constant1/1 -> Switch1/1
  Reset/1 -> Switch1/2
  In/1 -> Relational Operator/1
  Relational Operator/1 -> Switch2/1, Switch2/2
  max/1 -> Relational Operator/2

== system IRControlledSlidingDoor_Test/SignalProcessing/Counter/Latch2 ==
  In : Inport
  max : Inport  Port=2
  Reset : Inport  Port=3
  Constant1 : Constant  Value=0  OutDataTypeStr=boolean
  Relational Operator : RelationalOperator  OutDataTypeStr=boolean
  Switch1 : Switch  Criteria=u2 > Threshold
  Switch2 : Switch  Criteria=u2 > Threshold
  Unit Delay2 : UnitDelay  SampleTime=-1
  Out : Outport
  wires:
  Unit Delay2/1 -> Switch2/3
  Switch2/1 -> Switch1/3
  Switch1/1 -> Unit Delay2/1, Out/1
  Constant1/1 -> Switch1/1
  Reset/1 -> Switch1/2
  In/1 -> Relational Operator/1
  Relational Operator/1 -> Switch2/1, Switch2/2
  max/1 -> Relational Operator/2

== stateflow chart IRControlledSlidingDoor_Test/DoorOpening/Chart ==
  state A
  state B
  (default) -> A : {reopen=0;}
  A -> B : [close_initiated&&PIRSignal]{open_time = close_time;reopen=1;}
  B -> A : [close_cmplt]{reopen=0;}
  data: close_initiated input; PIRSignal input; close_time input; open_time output double; close_cmplt input; reopen output double
